simulink model "lunar_lander"  (R2019a)
settings: Solver=VariableStepAuto  StartTime=0.0  StopTime=100  RelTol=1e-3
values from neighbouring files (symbols this model uses):
  F_Thrust = 12500    [parameters.m]
  G = 6.6743e-11    [parameters.m]
  m_Impuls = 140    [parameters.m]
  m_Lunar_leer = 2134    [parameters.m]
  m_Mond = 7.346e22    (= 7.346e+22)    [parameters.m]
  m_Tank = 8200    [parameters.m]
  r_Mond = 1737000    [parameters.m]
  s_Lunar = sim.s_Lunar(time_idx)    [animate_result.m]    (also in parameters.m = 1000)
  v_Lunar = -60    [parameters.m]
libraries: simulink x3
settings Model: Creator=micha  LastModifiedBy=micha

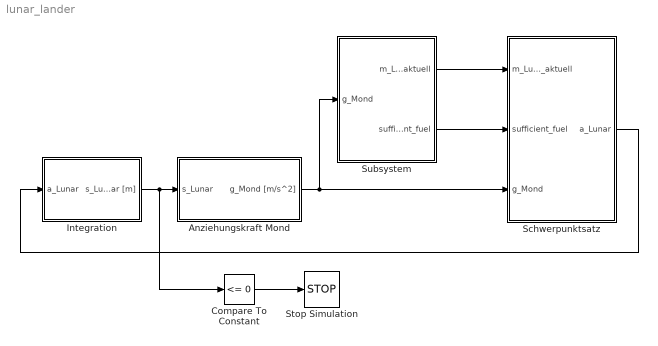
== system lunar_lander ==
  Anziehungskraft Mond : Subsystem
  Compare To Constant : simulink/Logic and Bit Operations/Compare To Constant  relop=<=  const=0  OutDataTypeStr=boolean
  Integration : Subsystem
  Schwerpunktsatz : Subsystem
  Stop Simulation : Stop
  Subsystem : Subsystem
  wires:
  Anziehungskraft Mond/1(g_Mond [m/s^2]) -> Subsystem/1(g_Mond), Schwerpunktsatz/3(g_Mond)
  Subsystem/1(m_Lunar_aktuell) -> Schwerpunktsatz/1(m_Lunar_aktuell)
  Schwerpunktsatz/1(a_Lunar) -> Integration/1(a_Lunar)
  Integration/1(s_Lunar [m]) -> Compare To Constant/1, Anziehungskraft Mond/1(s_Lunar)
  Compare To Constant/1 -> Stop Simulation/1
  Subsystem/2(sufficient_fuel) -> Schwerpunktsatz/2(sufficient_fuel)

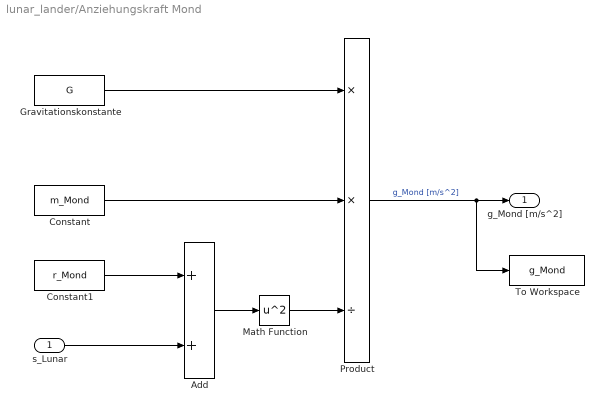
== system lunar_lander/Anziehungskraft Mond ==
  s_Lunar : Inport
  Add : Sum
  Constant : Constant  Value=m_Mond
  Constant1 : Constant  Value=r_Mond
  Gravitationskonstante : Constant  Value=G
  Math Function : Math  Operator=square  SaturateOnIntegerOverflow=on
  Product : Product  Inputs=**/
  To Workspace : ToWorkspace  VariableName=g_Mond  SaveFormat=Structure With Time  SampleTime=-1
  g_Mond [m/s^2] : Outport
  wires:
  Constant/1 -> Product/2
  s_Lunar/1 -> Add/2
  Add/1 -> Math Function/1
  Gravitationskonstante/1 -> Product/1
  Constant1/1 -> Add/1
  Math Function/1 -> Product/3
  Product/1 -> To Workspace/1, g_Mond [m/s^2]/1  "g_Mond [m/s^2]"

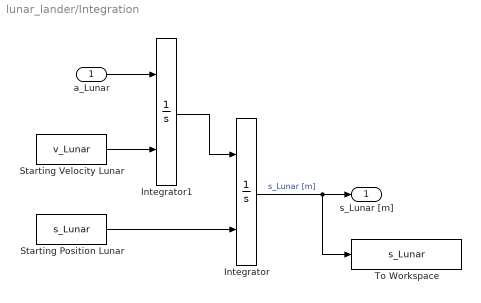
== system lunar_lander/Integration ==
  a_Lunar : Inport
  Integrator : Integrator  InitialConditionSource=external
  Integrator1 : Integrator  InitialConditionSource=external
  Starting Position Lunar : Constant  Value=s_Lunar
  Starting Velocity Lunar : Constant  Value=v_Lunar
  To Workspace : ToWorkspace  VariableName=s_Lunar  SaveFormat=Structure With Time  SampleTime=-1
  s_Lunar [m] : Outport
  wires:
  Integrator/1 -> s_Lunar [m]/1, To Workspace/1  "s_Lunar [m]"
  Integrator1/1 -> Integrator/1
  Starting Velocity Lunar/1 -> Integrator1/2
  a_Lunar/1 -> Integrator1/1
  Starting Position Lunar/1 -> Integrator/2

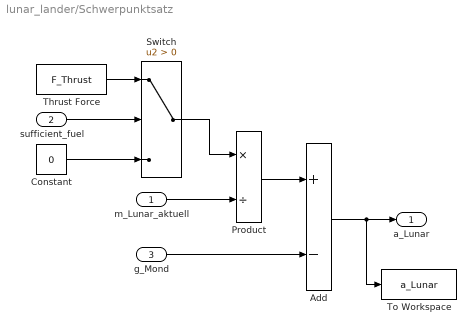
== system lunar_lander/Schwerpunktsatz ==
  m_Lunar_aktuell : Inport
  sufficient_fuel : Inport  Port=2
  g_Mond : Inport  Port=3
  Add : Sum  Inputs=+-
  Constant : Constant  Value=0
  Product : Product  Inputs=*/
  Switch : Switch  Criteria=u2 > Threshold
  Thrust Force : Constant  Value=F_Thrust
  To Workspace : ToWorkspace  VariableName=a_Lunar  SaveFormat=Structure With Time  SampleTime=-1
  a_Lunar : Outport
  wires:
  g_Mond/1 -> Add/2
  Add/1 -> To Workspace/1, a_Lunar/1
  m_Lunar_aktuell/1 -> Product/2
  Product/1 -> Add/1
  Thrust Force/1 -> Switch/1
  Switch/1 -> Product/1
  Constant/1 -> Switch/3
  sufficient_fuel/1 -> Switch/2

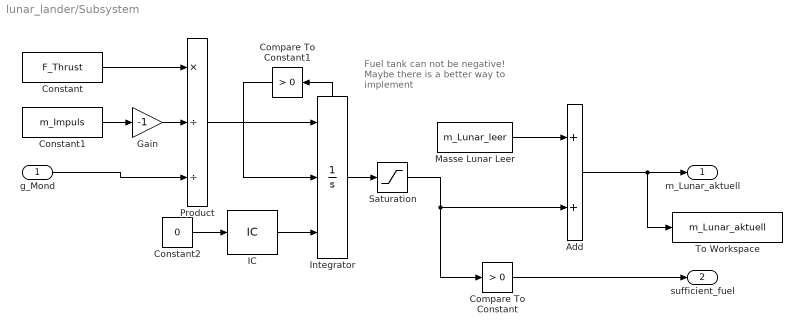
== system lunar_lander/Subsystem ==
  note: Fuel tank can not be negative!
      | Maybe there is a better way to implement
  g_Mond : Inport
  Add : Sum
  Compare To Constant : simulink/Logic and Bit Operations/Compare To Constant  relop=>  const=0  OutDataTypeStr=boolean
  Compare To Constant1 : simulink/Logic and Bit Operations/Compare To Constant  relop=>  const=0  OutDataTypeStr=boolean
  Constant : Constant  Value=F_Thrust
  Constant1 : Constant  Value=m_Impuls
  Constant2 : Constant  Value=0
  Gain : Gain  Gain=-1
  IC : InitialCondition  Value=m_Tank
  Integrator : Integrator  ExternalReset=either  InitialConditionSource=external  ShowStatePort=on
  Masse Lunar Leer : Constant  Value=m_Lunar_leer
  Product : Product  Inputs=*//
  Saturation : Saturate  UpperLimit=inf  LowerLimit=0
  To Workspace : ToWorkspace  VariableName=m_Lunar_aktuell  SaveFormat=Structure With Time  SampleTime=-1
  m_Lunar_aktuell : Outport
  sufficient_fuel : Outport  Port=2
  wires:
  IC/1 -> Integrator/3
  g_Mond/1 -> Product/3
  Constant/1 -> Product/1
  Constant1/1 -> Gain/1
  Product/1 -> Integrator/1
  Gain/1 -> Product/2
  Masse Lunar Leer/1 -> Add/1
  Add/1 -> To Workspace/1, m_Lunar_aktuell/1
  Integrator/1 -> Saturation/1
  Compare To Constant/1 -> sufficient_fuel/1
  Constant2/1 -> IC/1
  Integrator/State -> Compare To Constant1/1
  Compare To Constant1/1 -> Integrator/2
  Saturation/1 -> Compare To Constant/1, Add/2
